simulink model "EHB_MOTOR_r2018b"  (R2018b)
settings: Solver=FixedStepDiscrete  StartTime=0.0  StopTime=0.2  FixedStep=0.0001  RelTol=1e-3  EnableMultiTasking=on
undefined symbols (not defined in the file): CAN_EHB_VCU0x125, CAN_EHB_VCU0x126, CAN_id0x120_Data, Cos_Table, Cos_Table1, EHB_DTC_status, Sin_BreakPoint, Sin_BreakPoint1, Sin_Table, Sin_Table1
libraries: simulink x30
(part 2 of 7)

== system EHB_MOTOR_r2018b/EPB_CTRL/Subsystem1 ==
  Trigger : TriggerPort  TriggerType=function-call  VariantControl=Variant  PortDimensions=1
  Bus Creator : BusCreator  Inputs=11
  Data Store Memory11 : DataStoreMemory  DataStoreName=EPB_vBAT_AD  ReadBeforeWriteMsg=warning  WriteAfterWriteMsg=warning  WriteAfterReadMsg=warning  ShowAdditionalParam=off  OutDataTypeStr=uint16
      settings: RTWStateStorageClass=ExportedGlobal
  Data Store Memory12 : DataStoreMemory  DataStoreName=EPB1_Temp_AD  ReadBeforeWriteMsg=warning  WriteAfterWriteMsg=warning  WriteAfterReadMsg=warning  ShowAdditionalParam=off  OutDataTypeStr=uint16
      settings: RTWStateStorageClass=ExportedGlobal
  Data Store Memory13 : DataStoreMemory  DataStoreName=EPB_APBSwitch2_AD  ReadBeforeWriteMsg=warning  WriteAfterWriteMsg=warning  WriteAfterReadMsg=warning  ShowAdditionalParam=off  OutDataTypeStr=uint16
      settings: RTWStateStorageClass=ExportedGlobal
  Data Store Memory14 : DataStoreMemory  DataStoreName=EPB_7181PreDriver1_AD  ReadBeforeWriteMsg=warning  WriteAfterWriteMsg=warning  WriteAfterReadMsg=warning  ShowAdditionalParam=off  OutDataTypeStr=uint16
      settings: RTWStateStorageClass=ExportedGlobal
  Data Store Memory15 : DataStoreMemory  DataStoreName=EPB2_Temp_AD  ReadBeforeWriteMsg=warning  WriteAfterWriteMsg=warning  WriteAfterReadMsg=warning  ShowAdditionalParam=off  OutDataTypeStr=uint16
      settings: RTWStateStorageClass=ExportedGlobal
  Data Store Memory17 : DataStoreMemory  DataStoreName=EPB_APBSwitch3_AD  ReadBeforeWriteMsg=warning  WriteAfterWriteMsg=warning  WriteAfterReadMsg=warning  ShowAdditionalParam=off  OutDataTypeStr=uint16
      settings: RTWStateStorageClass=ExportedGlobal
  Data Store Memory18 : DataStoreMemory  DataStoreName=EPB_APBSwitch4_AD  ReadBeforeWriteMsg=warning  WriteAfterWriteMsg=warning  WriteAfterReadMsg=warning  ShowAdditionalParam=off  OutDataTypeStr=uint16
      settings: RTWStateStorageClass=ExportedGlobal
  Data Store Memory19 : DataStoreMemory  DataStoreName=EPB2_Current_AD  ReadBeforeWriteMsg=warning  WriteAfterWriteMsg=warning  WriteAfterReadMsg=warning  ShowAdditionalParam=off  OutDataTypeStr=uint16
      settings: RTWStateStorageClass=ExportedGlobal
  Data Store Memory20 : DataStoreMemory  DataStoreName=EPB_APBSwitch1_AD  ReadBeforeWriteMsg=warning  WriteAfterWriteMsg=warning  WriteAfterReadMsg=warning  ShowAdditionalParam=off  OutDataTypeStr=uint16
      settings: RTWStateStorageClass=ExportedGlobal
  Data Store Memory21 : DataStoreMemory  DataStoreName=EPB1_Current_AD  ReadBeforeWriteMsg=warning  WriteAfterWriteMsg=warning  WriteAfterReadMsg=warning  ShowAdditionalParam=off  OutDataTypeStr=uint16
      settings: RTWStateStorageClass=ExportedGlobal
  Data Store Memory22 : DataStoreMemory  DataStoreName=EPB_7181PreDriver2_AD  ReadBeforeWriteMsg=warning  WriteAfterWriteMsg=warning  WriteAfterReadMsg=warning  ShowAdditionalParam=off  OutDataTypeStr=uint16
      settings: RTWStateStorageClass=ExportedGlobal
  Data Store Read11 : DataStoreRead  DataStoreName=EPB_vBAT_AD  DataStoreElements=EPB_vBAT_AD
  Data Store Read12 : DataStoreRead  DataStoreName=EPB1_Temp_AD  DataStoreElements=EPB1_Temp_AD
  Data Store Read13 : DataStoreRead  DataStoreName=EPB_APBSwitch2_AD  DataStoreElements=EPB_APBSwitch2_AD
  Data Store Read14 : DataStoreRead  DataStoreName=EPB_7181PreDriver1_AD  DataStoreElements=EPB_7181PreDriver1_AD
  Data Store Read15 : DataStoreRead  DataStoreName=EPB2_Temp_AD  DataStoreElements=EPB2_Temp_AD
  Data Store Read17 : DataStoreRead  DataStoreName=EPB_APBSwitch3_AD  DataStoreElements=EPB_APBSwitch3_AD
  Data Store Read18 : DataStoreRead  DataStoreName=EPB_APBSwitch4_AD  DataStoreElements=EPB_APBSwitch4_AD
  Data Store Read19 : DataStoreRead  DataStoreName=EPB2_Current_AD  DataStoreElements=EPB2_Current_AD
  Data Store Read20 : DataStoreRead  DataStoreName=EPB_APBSwitch1_AD  DataStoreElements=EPB_APBSwitch1_AD
  Data Store Read21 : DataStoreRead  DataStoreName=EPB1_Current_AD  DataStoreElements=EPB1_Current_AD
  Data Store Read22 : DataStoreRead  DataStoreName=EPB_7181PreDriver2_AD  DataStoreElements=EPB_7181PreDriver2_AD
  EPB_interface : Subsystem
  EPB_INPUTBUS : Outport
  wires:
  Data Store Read21/1 -> EPB_interface/2(EPB1_Current_AD)
  Data Store Read17/1 -> EPB_interface/6(EPB_APBSwitch3_AD)
  Data Store Read14/1 -> EPB_interface/11(EPB_7181PreDriver1_AD)
  Data Store Read13/1 -> EPB_interface/10(EPB_7181PreDriver2_AD)
  EPB_interface/9(EPB_APBSwitch2_filtered) -> Bus Creator/9  "EPB_7181PreDriver2_filtered"
  Data Store Read19/1 -> EPB_interface/3(EPB2_Current_AD)
  Data Store Read12/1 -> EPB_interface/4(EPB1_Temp_AD)
  Data Store Read22/1 -> EPB_interface/9(EPB_APBSwitch2_AD)
  Data Store Read15/1 -> EPB_interface/5(EPB2_Temp_AD)
  Data Store Read20/1 -> EPB_interface/8(EPB_APBSwitch1_AD)
  EPB_interface/7(EPB_APBSwitch4_filtered) -> Bus Creator/7  "EPB_APBSwitch4_filtered"
  EPB_interface/11(EPB_7181PreDriver1_filtered) -> Bus Creator/11  "EPB_7181PreDriver1_filtered"
  EPB_interface/4(EPB1_Temp) -> Bus Creator/4  "EPB1_Temp"
  EPB_interface/3(EPB2_Current_filtered) -> Bus Creator/3  "EPB2_Current_filtered"
  Data Store Read11/1 -> EPB_interface/1(EPB_vBAT_AD)
  EPB_interface/2(EPB1_Current_filtered) -> Bus Creator/2  "EPB1_Current_filtered"
  Data Store Read18/1 -> EPB_interface/7(EPB_APBSwitch4_AD)
  EPB_interface/6(EPB_APBSwitch3_filtered) -> Bus Creator/6  "EPB_APBSwitch3_filtered"
  EPB_interface/5(EPB2_Temp) -> Bus Creator/5  "EPB2_Temp"
  EPB_interface/1(EPB_vBAT_filtered) -> Bus Creator/1  "EPB_vBAT_filtered"
  EPB_interface/10(EPB_7181PreDriver2_filtered) -> Bus Creator/10  "EPB_APBSwitch2_filtered"
  EPB_interface/8(EPB_APBSwitch1_filtered) -> Bus Creator/8  "EPB_APBSwitch1_filtered"
  Bus Creator/1 -> EPB_INPUTBUS/1

== system EHB_MOTOR_r2018b/EHB_MOTOR_PRO/DIAG/5vDiag ==
  note: 20ms
  note: 5v输出异常
  5vVoltage : Inport
  Chart : Stateflow chart  TreatAsAtomicUnit=on
  Subsystem : Subsystem
  5vErr : Outport
  wires:
  5vVoltage/1 -> Subsystem/1(In1)
  Subsystem/1(Out1) -> 5vErr/1
  Chart/1(task_20ms()) -> Subsystem/Trigger

== system EHB_MOTOR_r2018b/EHB_MOTOR_PRO/DIAG/AngleSensorDiag ==
  note: 角度传感器缺少标定
  note: 角度传感器没有信号
  note: 200ms
  note: 角度传感器信号超限故障
  note: 200ms
  note: 200ms
  AngleSensorSignal : Inport
  AngleSensorCalFlag : Inport  Port=2
  Chart : Stateflow chart  TreatAsAtomicUnit=on
  Chart1 : Stateflow chart  TreatAsAtomicUnit=on
  Chart2 : Stateflow chart  TreatAsAtomicUnit=on
  Subsystem : Subsystem
  Subsystem1 : Subsystem
  Subsystem2 : Subsystem
  AngleSensorSignalOverride : Outport
  AngleSensorSignalLost : Outport  Port=2
  AngleSensorNoCal : Outport  Port=3
  wires:
  Subsystem/1(Out1) -> AngleSensorSignalOverride/1
  Chart/1(task_200ms()) -> Subsystem/Trigger
  Chart1/1(task_200ms()) -> Subsystem1/Trigger
  Subsystem1/1(Out1) -> AngleSensorSignalLost/1
  AngleSensorSignal/1 -> Subsystem1/1(In1), Subsystem/1(In1)
  Subsystem2/1(Out1) -> AngleSensorNoCal/1
  Chart2/1(task_200ms()) -> Subsystem2/Trigger
  AngleSensorCalFlag/1 -> Subsystem2/1(In1)

== system EHB_MOTOR_r2018b/EHB_MOTOR_PRO/DIAG/BusOffDiag ==
  note: 控制器内部故障
  In1 : Inport
  Ground : Ground
  Terminator : Terminator
  BusOffErr : Outport
  wires:
  In1/1 -> Terminator/1
  Ground/1 -> BusOffErr/1

== system EHB_MOTOR_r2018b/EHB_MOTOR_PRO/DIAG/CANCommDiag ==
  note: CAN收发模块故障
  In1 : Inport
  Ground : Ground
  Terminator : Terminator
  CANCommErr : Outport
  wires:
  In1/1 -> Terminator/1
  Ground/1 -> CANCommErr/1

== system EHB_MOTOR_r2018b/EHB_MOTOR_PRO/DIAG/CANDataLostDiag ==
  note: CAN丢失数据
  In1 : Inport
  Ground : Ground
  Terminator : Terminator
  CANDataLostErr : Outport
  wires:
  In1/1 -> Terminator/1
  Ground/1 -> CANDataLostErr/1

== system EHB_MOTOR_r2018b/EHB_MOTOR_PRO/DIAG/Chip7189Diag ==
  note: 7189芯片故障
  note: 20ms
  Chart : Stateflow chart  TreatAsAtomicUnit=on
  Data Store Memory1 : DataStoreMemory  DataStoreName=Chip7189ErrFlag  ReadBeforeWriteMsg=warning  WriteAfterWriteMsg=warning  WriteAfterReadMsg=warning  ShowAdditionalParam=off  OutDataTypeStr=uint8
      settings: RTWStateStorageClass=ExportedGlobal
  Data Store Read2 : DataStoreRead  DataStoreName=Chip7189ErrFlag  DataStoreElements=Chip7189ErrFlag
  Subsystem : Subsystem
  Chip7189_err : Outport
  wires:
  Chart/1(task_20ms()) -> Subsystem/Trigger
  Subsystem/1(Out1) -> Chip7189_err/1
  Data Store Read2/1 -> Subsystem/1(In1)

== system EHB_MOTOR_r2018b/EHB_MOTOR_PRO/DIAG/CurrentSensorDiag ==
  note: 200ms
  note: U相电流传感器故障
  note: 200ms
  note: V相电流传感器故障
  note: 200ms
  note: W相电流传感器故障
  CurrentSensorU : Inport
  CurrentSensorV : Inport  Port=2
  CurrentSensorW : Inport  Port=3
  Chart : Stateflow chart  TreatAsAtomicUnit=on
  Chart1 : Stateflow chart  TreatAsAtomicUnit=on
  Chart2 : Stateflow chart  TreatAsAtomicUnit=on
  Subsystem : Subsystem
  Subsystem1 : Subsystem
  Subsystem2 : Subsystem
  CurrentSensorUOverride : Outport
  CurrentSensorVOverride : Outport  Port=2
  CurrentSensorWOverride : Outport  Port=3
  wires:
  CurrentSensorU/1 -> Subsystem/1(In1)
  Subsystem/1(Out1) -> CurrentSensorUOverride/1
  Chart/1(task_200ms()) -> Subsystem/Trigger
  Chart1/1(task_200ms()) -> Subsystem1/Trigger
  Subsystem1/1(Out1) -> CurrentSensorVOverride/1
  CurrentSensorV/1 -> Subsystem1/1(In1)
  CurrentSensorW/1 -> Subsystem2/1(In1)
  Subsystem2/1(Out1) -> CurrentSensorWOverride/1
  Chart2/1(task_200ms()) -> Subsystem2/Trigger

== system EHB_MOTOR_r2018b/EHB_MOTOR_PRO/DIAG/EHBDiag ==
  note: EHB电源电压过高
  note: 200ms
  note: EHB电源电压过低
  EHBVoltage : Inport
  Chart : Stateflow chart  TreatAsAtomicUnit=on
  Subsystem : Subsystem
  EHBVoltageLow1 : Outport
  EHBVoltageLow2 : Outport  Port=2
  EHBVoltageHigh1 : Outport  Port=3
  EHBVoltageHigh2 : Outport  Port=4
  wires:
  EHBVoltage/1 -> Subsystem/1(In1)
  Subsystem/1(EHBVoltageLow1) -> EHBVoltageLow1/1
  Chart/1(task_200ms()) -> Subsystem/Trigger
  Subsystem/3(EHBVoltageHigh1) -> EHBVoltageHigh1/1
  Subsystem/2(EHBVoltageLow2) -> EHBVoltageLow2/1
  Subsystem/4(EHBVoltageHigh2) -> EHBVoltageHigh2/1

== system EHB_MOTOR_r2018b/EHB_MOTOR_PRO/DIAG/KL15VoltageDiag ==
  note: KL15电压过低
  note: 200ms
  note: KL15电压过高
  KL15Voltage : Inport
  Chart : Stateflow chart  TreatAsAtomicUnit=on
  Subsystem : Subsystem
  KL15VoltageLow : Outport
  KL15VoltageHigh : Outport  Port=2
  wires:
  Subsystem/2(Out2) -> KL15VoltageHigh/1
  Chart/1(task_200ms()) -> Subsystem/Trigger
  Subsystem/1(Out1) -> KL15VoltageLow/1
  KL15Voltage/1 -> Subsystem/1(In1)

== system EHB_MOTOR_r2018b/EHB_MOTOR_PRO/DIAG/LogicVoltageDiag ==
  note: 12VLogic电源电压过高
  note: 200ms
  note: 12VLogic电源电压过低
  LogicVoltage : Inport
  Chart : Stateflow chart  TreatAsAtomicUnit=on
  Subsystem : Subsystem
  LogicVoltageLow : Outport
  LogicVoltageHigh : Outport  Port=2
  wires:
  LogicVoltage/1 -> Subsystem/1(In1)
  Subsystem/1(Out1) -> LogicVoltageLow/1
  Chart/1(task_200ms()) -> Subsystem/Trigger
  Subsystem/2(Out2) -> LogicVoltageHigh/1

== system EHB_MOTOR_r2018b/EHB_MOTOR_PRO/DIAG/MotLockDiag ==
  In1 : Inport
  Abs : Abs
  Abs1 : Abs
  Abs2 : Abs
  Bus Selector : BusSelector  OutputSignals=Feedback.TEMP_DELAY.EHB_Mot_length,AI_BUS.EHB_iU_filtered,AI_BUS.EHB_iV_filtered,AI_BUS.EHB_iW_filtered
  Constant : Constant  Value=2
  Constant1 : Constant  Value=70
  Constant2 : Constant  Value=70
  Constant3 : Constant  Value=70
  Constant4 : Constant  Value=0  OutDataTypeStr=uint8
  Data Store Memory1 : DataStoreMemory  DataStoreName=tiMotLocked_C  ReadBeforeWriteMsg=warning  WriteAfterWriteMsg=warning  WriteAfterReadMsg=warning  ShowAdditionalParam=off  OutDataTypeStr=uint16
      settings: RTWStateStorageClass=ExportedGlobal
  Data Store Read : DataStoreRead  DataStoreName=tiMotLocked_C  DataStoreElements=tiMotLocked_C
  ErrorSignalCount : Stateflow chart  TreatAsAtomicUnit=on
  Logical Operator : Logic  Operator=OR  Inputs=3  AllPortsSameDT=off  OutDataTypeStr=boolean
  Logical Operator1 : Logic  AllPortsSameDT=off  OutDataTypeStr=boolean
  Relational Operator : RelationalOperator  Operator=<  OutDataTypeStr=boolean  RndMeth=Simplest
  Relational Operator1 : RelationalOperator  Operator=>  OutDataTypeStr=boolean  RndMeth=Simplest
  Relational Operator2 : RelationalOperator  Operator=>  OutDataTypeStr=boolean  RndMeth=Simplest
  Relational Operator3 : RelationalOperator  Operator=>  OutDataTypeStr=boolean  RndMeth=Simplest
  Mot_locked_err : Outport
  wires:
  In1/1 -> Bus Selector/1
  Bus Selector/1 -> Relational Operator/1  "<EHB_Mot_length>"
  Constant/1 -> Relational Operator/2
  Constant1/1 -> Relational Operator1/2
  Bus Selector/2 -> Abs/1  "<EHB_iU_filtered>"
  Constant2/1 -> Relational Operator2/2
  Constant3/1 -> Relational Operator3/2
  Bus Selector/4 -> Abs2/1  "<EHB_iW_filtered>"
  Bus Selector/3 -> Abs1/1  "<EHB_iV_filtered>"
  Relational Operator1/1 -> Logical Operator/1
  Relational Operator2/1 -> Logical Operator/2
  Relational Operator3/1 -> Logical Operator/3
  Logical Operator/1 -> Logical Operator1/2
  Relational Operator/1 -> Logical Operator1/1
  Logical Operator1/1 -> ErrorSignalCount/1(Mot_locked)
  Abs/1 -> Relational Operator1/1
  Abs1/1 -> Relational Operator2/1
  Abs2/1 -> Relational Operator3/1
  Constant4/1 -> ErrorSignalCount/3(Recover)
  ErrorSignalCount/1(Mot_locked_err) -> Mot_locked_err/1
  Data Store Read/1 -> ErrorSignalCount/2(tiMotLocked_C)

== system EHB_MOTOR_r2018b/EHB_MOTOR_PRO/DIAG/MotorDiag ==
  note: 200ms
  note: 电机回路故障
  note: 200ms
  note: 电机过温
  note: 电机过流故障
  note: 200ms
  MotorCircuitCurrent : Inport
  Motor_PWMout : Inport  Port=2
  MotorTemp : Inport  Port=3
  MotorCurrent : Inport  Port=4
  Chart : Stateflow chart  TreatAsAtomicUnit=on
  Chart1 : Stateflow chart  TreatAsAtomicUnit=on
  Chart2 : Stateflow chart  TreatAsAtomicUnit=on
  Subsystem : Subsystem
  Subsystem1 : Subsystem
  Subsystem2 : Subsystem
  MotorCircuitCurrentOverride : Outport
  MotorTempOverride : Outport  Port=2
  MotorCurrentOverride : Outport  Port=3
  wires:
  Subsystem1/1(Out1) -> MotorTempOverride/1
  Chart1/1(task_200ms()) -> Subsystem1/Trigger
  Chart/1(task_200ms()) -> Subsystem/Trigger
  Subsystem/1(Out1) -> MotorCircuitCurrentOverride/1
  MotorCircuitCurrent/1 -> Subsystem/1(In1)
  MotorTemp/1 -> Subsystem1/1(In1)
  MotorCurrent/1 -> Subsystem2/1(In1)
  Subsystem2/1(Out1) -> MotorCurrentOverride/1
  Chart2/1(task_200ms()) -> Subsystem2/Trigger
  Motor_PWMout/1 -> Subsystem/2(Motor_PWMout)

== system EHB_MOTOR_r2018b/EHB_MOTOR_PRO/DIAG/PWMCircuitDiag ==
  note: PWM波发送电路故障
  In1 : Inport
  Ground : Ground
  Terminator : Terminator
  PWMCircuitErr : Outport
  wires:
  In1/1 -> Terminator/1
  Ground/1 -> PWMCircuitErr/1

== system EHB_MOTOR_r2018b/EHB_MOTOR_PRO/DIAG/PressureSensorDiag ==
  note: 200ms
  note: 200ms
  note: 压力跟随故障
  note: 200ms
  note: 压力传感器故障
  note: 压力传感器缺少标定
  VCU_Brake_AimPressure : Inport
  EHB_actPresure_filtered : Inport  Port=2
  EHB_Presure_ADC : Inport  Port=3
  PressureSensorCalFlag : Inport  Port=4
  Chart : Stateflow chart  TreatAsAtomicUnit=on
  Chart1 : Stateflow chart  TreatAsAtomicUnit=on
  Chart2 : Stateflow chart  TreatAsAtomicUnit=on
  Subsystem : Subsystem
  Subsystem1 : Subsystem
  Subsystem2 : Subsystem
  PressureFlowERR1 : Outport
  PressureFlowERR2 : Outport  Port=2
  PressureSensorERR : Outport  Port=3
  PressureSensorNoCal : Outport  Port=4
  wires:
  Chart2/1(task_200ms()) -> Subsystem2/Trigger
  Subsystem2/1(Out1) -> PressureSensorNoCal/1
  EHB_actPresure_filtered/1 -> Subsystem/2(EHB_actPresure_filtered)
  Subsystem1/1(Out1) -> PressureSensorERR/1
  Chart1/1(task_200ms()) -> Subsystem1/Trigger
  Chart/1(task_200ms()) -> Subsystem/Trigger
  Subsystem/1(Out1) -> PressureFlowERR1/1
  PressureSensorCalFlag/1 -> Subsystem2/1(In1)
  VCU_Brake_AimPressure/1 -> Subsystem/1(VCU_Brake_AimPressure)
  Subsystem/2(Out2) -> PressureFlowERR2/1
  EHB_Presure_ADC/1 -> Subsystem1/1(EHB_Presure_ADC)

== system EHB_MOTOR_r2018b/EHB_MOTOR_PRO/DIAG/RespondOvertimeDiag ==
  note: 响应超时故障
  In1 : Inport
  Ground : Ground
  Terminator : Terminator
  Chip7189_err : Outport
  wires:
  Ground/1 -> Chip7189_err/1
  In1/1 -> Terminator/1

== system EHB_MOTOR_r2018b/EHB_MOTOR_PRO/DIAG/SpeedSensorDiag ==
  note: 200ms
  note: 轮速传感器信号电压异常
  SpeedSensor : Inport
  Chart : Stateflow chart  TreatAsAtomicUnit=on
  Subsystem : Subsystem
  SpeedSensorOverride : Outport
  wires:
  SpeedSensor/1 -> Subsystem/1(In1)
  Chart/1(task_200ms()) -> Subsystem/Trigger
  Subsystem/1(Out1) -> SpeedSensorOverride/1

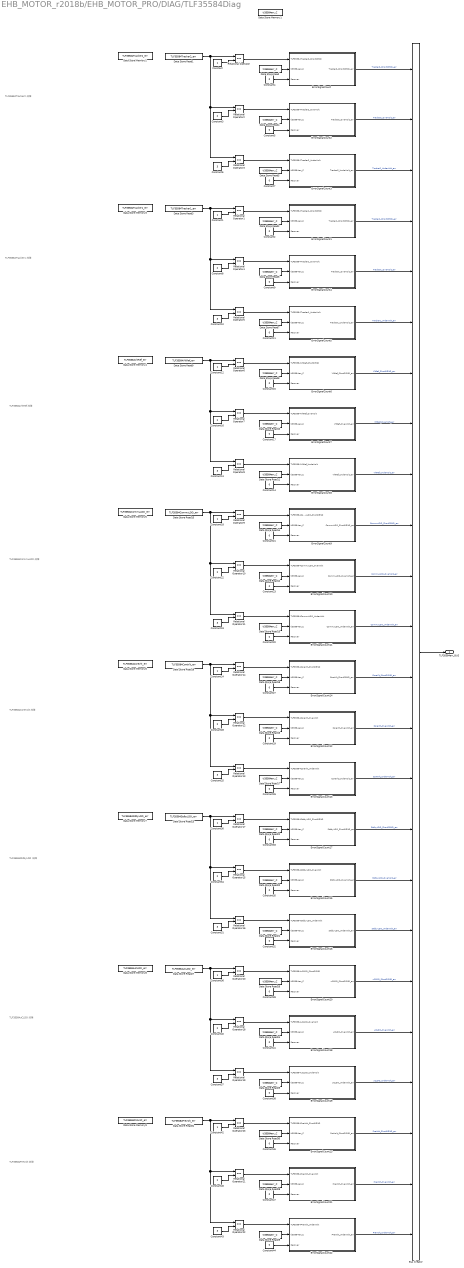
== system EHB_MOTOR_r2018b/EHB_MOTOR_PRO/DIAG/TLF35584Diag ==
  note: TLF35584Tracker2故障
  note: TLF35584Tracker1故障
  note: TLF35584VltRef故障
  note: TLF35584CommuLDO故障
  note: TLF35584CoreVolt故障
  note: TLF35584StdbyLDO故障
  note: TLF35584uCLDO故障
  note: TLF35584PreVolt故障
  Bus Creator : BusCreator  Inputs=24
  Constant{,1,12,18,24,30,36,42} (8 alike) : Constant
  Constant{6,10,13,19,25,31,37,43} (8 alike) : Constant  Value=3
  Constant{2,4..5,7,9,11,14..15,17,20..21,23,26..27,29,32..33,35,38..39,41,44..45,47} (24 alike) : Constant  Value=0  OutDataTypeStr=uint8
  Constant{3,8,16,22,28,34,40,46} (8 alike) : Constant  Value=2
  Data Store Memory1 : DataStoreMemory  DataStoreName=ti35584err_C  ReadBeforeWriteMsg=warning  WriteAfterWriteMsg=warning  WriteAfterReadMsg=warning  ShowAdditionalParam=off  OutDataTypeStr=uint16
      settings: RTWStateStorageClass=ExportedGlobal
  Data Store Memory2 : DataStoreMemory  DataStoreName=TLF35584Tracker2_err  ReadBeforeWriteMsg=warning  WriteAfterWriteMsg=warning  WriteAfterReadMsg=warning  ShowAdditionalParam=off  OutDataTypeStr=uint8
      settings: RTWStateStorageClass=ExportedGlobal
  Data Store Memory3 : DataStoreMemory  DataStoreName=TLF35584Tracker1_err  ReadBeforeWriteMsg=warning  WriteAfterWriteMsg=warning  WriteAfterReadMsg=warning  ShowAdditionalParam=off  OutDataTypeStr=uint8
      settings: RTWStateStorageClass=ExportedGlobal
  Data Store Memory4 : DataStoreMemory  DataStoreName=TLF35584VltRef_err  ReadBeforeWriteMsg=warning  WriteAfterWriteMsg=warning  WriteAfterReadMsg=warning  ShowAdditionalParam=off  OutDataTypeStr=uint8
      settings: RTWStateStorageClass=ExportedGlobal
  Data Store Memory5 : DataStoreMemory  DataStoreName=TLF35584CommuLDO_err  ReadBeforeWriteMsg=warning  WriteAfterWriteMsg=warning  WriteAfterReadMsg=warning  ShowAdditionalParam=off  OutDataTypeStr=uint8
      settings: RTWStateStorageClass=ExportedGlobal
  Data Store Memory6 : DataStoreMemory  DataStoreName=TLF35584CoreVlt_err  ReadBeforeWriteMsg=warning  WriteAfterWriteMsg=warning  WriteAfterReadMsg=warning  ShowAdditionalParam=off  OutDataTypeStr=uint8
      settings: RTWStateStorageClass=ExportedGlobal
  Data Store Memory7 : DataStoreMemory  DataStoreName=TLF35584StdbyLDO_err  ReadBeforeWriteMsg=warning  WriteAfterWriteMsg=warning  WriteAfterReadMsg=warning  ShowAdditionalParam=off  OutDataTypeStr=uint8
      settings: RTWStateStorageClass=ExportedGlobal
  Data Store Memory8 : DataStoreMemory  DataStoreName=TLF35584uCLDO_err  ReadBeforeWriteMsg=warning  WriteAfterWriteMsg=warning  WriteAfterReadMsg=warning  ShowAdditionalParam=off  OutDataTypeStr=uint8
      settings: RTWStateStorageClass=ExportedGlobal
  Data Store Memory9 : DataStoreMemory  DataStoreName=TLF35584PreVolt_err  ReadBeforeWriteMsg=warning  WriteAfterWriteMsg=warning  WriteAfterReadMsg=warning  ShowAdditionalParam=off  OutDataTypeStr=uint8
      settings: RTWStateStorageClass=ExportedGlobal
  Data Store Read{,2,4..8,10..14,16..18,20..22,24..26,28..30} (24 alike) : DataStoreRead  DataStoreName=ti35584err_C  DataStoreElements=ti35584err_C
  Data Store Read1 : DataStoreRead  DataStoreName=TLF35584Tracker2_err  DataStoreElements=TLF35584Tracker2_err
  Data Store Read15 : DataStoreRead  DataStoreName=TLF35584CommuLDO_err  DataStoreElements=TLF35584CommuLDO_err
  Data Store Read19 : DataStoreRead  DataStoreName=TLF35584CoreVlt_err  DataStoreElements=TLF35584CoreVlt_err
  Data Store Read23 : DataStoreRead  DataStoreName=TLF35584StdbyLDO_err  DataStoreElements=TLF35584StdbyLDO_err
  Data Store Read27 : DataStoreRead  DataStoreName=TLF35584uCLDO_err  DataStoreElements=TLF35584uCLDO_err
  Data Store Read3 : DataStoreRead  DataStoreName=TLF35584Tracker1_err  DataStoreElements=TLF35584Tracker1_err
  Data Store Read31 : DataStoreRead  DataStoreName=TLF35584PreVolt_err  DataStoreElements=TLF35584PreVolt_err
  Data Store Read9 : DataStoreRead  DataStoreName=TLF35584VltRef_err  DataStoreElements=TLF35584VltRef_err
  ErrorSignalCount : Stateflow chart  TreatAsAtomicUnit=on
  ErrorSignalCount1 : Stateflow chart  TreatAsAtomicUnit=on
  ErrorSignalCount10 : Stateflow chart  TreatAsAtomicUnit=on
  ErrorSignalCount11 : Stateflow chart  TreatAsAtomicUnit=on
  ErrorSignalCount12 : Stateflow chart  TreatAsAtomicUnit=on
  ErrorSignalCount13 : Stateflow chart  TreatAsAtomicUnit=on
  ErrorSignalCount14 : Stateflow chart  TreatAsAtomicUnit=on
  ErrorSignalCount15 : Stateflow chart  TreatAsAtomicUnit=on
  ErrorSignalCount16 : Stateflow chart  TreatAsAtomicUnit=on
  ErrorSignalCount17 : Stateflow chart  TreatAsAtomicUnit=on
  ErrorSignalCount18 : Stateflow chart  TreatAsAtomicUnit=on
  ErrorSignalCount19 : Stateflow chart  TreatAsAtomicUnit=on
  ErrorSignalCount2 : Stateflow chart  TreatAsAtomicUnit=on
  ErrorSignalCount20 : Stateflow chart  TreatAsAtomicUnit=on
  ErrorSignalCount21 : Stateflow chart  TreatAsAtomicUnit=on
  ErrorSignalCount22 : Stateflow chart  TreatAsAtomicUnit=on
  ErrorSignalCount23 : Stateflow chart  TreatAsAtomicUnit=on
  ErrorSignalCount3 : Stateflow chart  TreatAsAtomicUnit=on
  ErrorSignalCount4 : Stateflow chart  TreatAsAtomicUnit=on
  ErrorSignalCount5 : Stateflow chart  TreatAsAtomicUnit=on
  ErrorSignalCount6 : Stateflow chart  TreatAsAtomicUnit=on
  ErrorSignalCount7 : Stateflow chart  TreatAsAtomicUnit=on
  ErrorSignalCount8 : Stateflow chart  TreatAsAtomicUnit=on
  ErrorSignalCount9 : Stateflow chart  TreatAsAtomicUnit=on
  Relational Operator{,1..23} (24 alike) : RelationalOperator  Operator===  OutDataTypeStr=boolean  RndMeth=Simplest
  TLF35584err_BUS : Outport
  wires:
  Data Store Read/1 -> ErrorSignalCount/2(ti35584err_C)
  Constant4/1 -> ErrorSignalCount/3(Recover)
  Data Store Read1/1 -> Relational Operator/1, Relational Operator2/1, Relational Operator3/1
  Constant/1 -> Relational Operator/2
  Relational Operator/1 -> ErrorSignalCount/1(TLF35584Tracker2_Short2GND)
  Relational Operator1/1 -> ErrorSignalCount1/1(TLF35584Tracker1_Short2GND)
  Constant1/1 -> Relational Operator1/2
  Constant2/1 -> ErrorSignalCount1/3(Recover)
  Data Store Read2/1 -> ErrorSignalCount1/2(ti35584err_C)
  Constant3/1 -> Relational Operator2/2
  Constant5/1 -> ErrorSignalCount2/3(Recover)
  Data Store Read4/1 -> ErrorSignalCount2/2(ti35584err_C)
  Relational Operator2/1 -> ErrorSignalCount2/1(TLF35584Tracker2_OverVolt)
  Constant6/1 -> Relational Operator3/2
  Relational Operator3/1 -> ErrorSignalCount3/1(TLF35584Tracker2_UnderVolt)
  Data Store Read5/1 -> ErrorSignalCount3/2(ti35584err_C)
  Constant7/1 -> ErrorSignalCount3/3(Recover)
  Constant11/1 -> ErrorSignalCount5/3(Recover)
  Data Store Read7/1 -> ErrorSignalCount5/2(ti35584err_C)
  Relational Operator5/1 -> ErrorSignalCount5/1(TLF35584Tracker1_UnderVolt)
  Constant10/1 -> Relational Operator5/2
  Relational Operator4/1 -> ErrorSignalCount4/1(TLF35584Tracker1_OverVolt)
  Data Store Read6/1 -> ErrorSignalCount4/2(ti35584err_C)
  Constant9/1 -> ErrorSignalCount4/3(Recover)
  Constant8/1 -> Relational Operator4/2
  Data Store Read3/1 -> Relational Operator5/1, Relational Operator4/1, Relational Operator1/1
  Data Store Read9/1 -> Relational Operator6/1, Relational Operator7/1, Relational Operator8/1
  Constant16/1 -> Relational Operator7/2
  Constant17/1 -> ErrorSignalCount7/3(Recover)
  Data Store Read10/1 -> ErrorSignalCount7/2(ti35584err_C)
  Relational Operator7/1 -> ErrorSignalCount7/1(TLF35584VltRef_OverVolt)
  Constant13/1 -> Relational Operator8/2
  Relational Operator8/1 -> ErrorSignalCount8/1(TLF35584VltRef_UnderVolt)
  Data Store Read11/1 -> ErrorSignalCount8/2(ti35584err_C)
  Constant14/1 -> ErrorSignalCount8/3(Recover)
  Data Store Read8/1 -> ErrorSignalCount6/2(ti35584err_C)
  Constant15/1 -> ErrorSignalCount6/3(Recover)
  Constant12/1 -> Relational Operator6/2
  Relational Operator6/1 -> ErrorSignalCount6/1(TLF35584VltRef_Short2GND)
  Relational Operator9/1 -> ErrorSignalCount9/1(TLF35584CommuLDO_Short2GND)
  Constant18/1 -> Relational Operator9/2
  Constant21/1 -> ErrorSignalCount9/3(Recover)
  Data Store Read14/1 -> ErrorSignalCount9/2(ti35584err_C)
  Constant20/1 -> ErrorSignalCount11/3(Recover)
  Data Store Read13/1 -> ErrorSignalCount11/2(ti35584err_C)
  Relational Operator11/1 -> ErrorSignalCount11/1(TLF35584CommuLDO_UnderVolt)
  Constant19/1 -> Relational Operator11/2
  Relational Operator10/1 -> ErrorSignalCount10/1(TLF35584CommuLDO_OverVolt)
  Data Store Read12/1 -> ErrorSignalCount10/2(ti35584err_C)
  Constant23/1 -> ErrorSignalCount10/3(Recover)
  Constant22/1 -> Relational Operator10/2
  Data Store Read15/1 -> Relational Operator11/1, Relational Operator10/1, Relational Operator9/1
  Data Store Read19/1 -> Relational Operator14/1, Relational Operator13/1, Relational Operator12/1
  Constant28/1 -> Relational Operator12/2
  Constant29/1 -> ErrorSignalCount12/3(Recover)
  Data Store Read16/1 -> ErrorSignalCount12/2(ti35584err_C)
  Relational Operator12/1 -> ErrorSignalCount12/1(TLF35584CoreVlt_OverVolt)
  Constant25/1 -> Relational Operator13/2
  Relational Operator13/1 -> ErrorSignalCount13/1(TLF35584CoreVlt_UnderVolt)
  Data Store Read17/1 -> ErrorSignalCount13/2(ti35584err_C)
  Constant26/1 -> ErrorSignalCount13/3(Recover)
  Data Store Read18/1 -> ErrorSignalCount14/2(ti35584err_C)
  Constant27/1 -> ErrorSignalCount14/3(Recover)
  Constant24/1 -> Relational Operator14/2
  Relational Operator14/1 -> ErrorSignalCount14/1(TLF35584CoreVlt_Short2GND)
  Relational Operator17/1 -> ErrorSignalCount17/1(TLF35584StdbyLDO_Short2GND)
  Constant30/1 -> Relational Operator17/2
  Constant33/1 -> ErrorSignalCount17/3(Recover)
  Data Store Read22/1 -> ErrorSignalCount17/2(ti35584err_C)
  Constant32/1 -> ErrorSignalCount16/3(Recover)
  Data Store Read21/1 -> ErrorSignalCount16/2(ti35584err_C)
  Relational Operator16/1 -> ErrorSignalCount16/1(TLF35584StdbyLDO_UnderVolt)
  Constant31/1 -> Relational Operator16/2
  Relational Operator15/1 -> ErrorSignalCount15/1(TLF35584StdbyLDO_OverVolt)
  Data Store Read20/1 -> ErrorSignalCount15/2(ti35584err_C)
  Constant35/1 -> ErrorSignalCount15/3(Recover)
  Constant34/1 -> Relational Operator15/2
  Data Store Read23/1 -> Relational Operator16/1, Relational Operator15/1, Relational Operator17/1
  Data Store Read27/1 -> Relational Operator20/1, Relational Operator19/1, Relational Operator18/1
  Constant40/1 -> Relational Operator18/2
  Constant41/1 -> ErrorSignalCount18/3(Recover)
  Data Store Read24/1 -> ErrorSignalCount18/2(ti35584err_C)
  Relational Operator18/1 -> ErrorSignalCount18/1(TLF35584uCLDO_OverVolt)
  Constant37/1 -> Relational Operator19/2
  Relational Operator19/1 -> ErrorSignalCount19/1(TLF35584uCLDO_UnderVolt)
  Data Store Read25/1 -> ErrorSignalCount19/2(ti35584err_C)
  Constant38/1 -> ErrorSignalCount19/3(Recover)
  Data Store Read26/1 -> ErrorSignalCount20/2(ti35584err_C)
  Constant39/1 -> ErrorSignalCount20/3(Recover)
  Constant36/1 -> Relational Operator20/2
  Relational Operator20/1 -> ErrorSignalCount20/1(TLF35584uCLDO_Short2GND)
  Relational Operator23/1 -> ErrorSignalCount23/1(TLF35584PreVolt_Short2GND)
  Constant42/1 -> Relational Operator23/2
  Constant45/1 -> ErrorSignalCount23/3(Recover)
  Data Store Read30/1 -> ErrorSignalCount23/2(ti35584err_C)
  Constant44/1 -> ErrorSignalCount22/3(Recover)
  Data Store Read29/1 -> ErrorSignalCount22/2(ti35584err_C)
  Relational Operator22/1 -> ErrorSignalCount22/1(TLF35584PreVolt_UnderVolt)
  Constant43/1 -> Relational Operator22/2
  Relational Operator21/1 -> ErrorSignalCount21/1(TLF35584PreVolt_OverVolt)
  Data Store Read28/1 -> ErrorSignalCount21/2(ti35584err_C)
  Constant47/1 -> ErrorSignalCount21/3(Recover)
  Constant46/1 -> Relational Operator21/2
  Data Store Read31/1 -> Relational Operator22/1, Relational Operator21/1, Relational Operator23/1
  ErrorSignalCount/1(Tracker2_Short2GND_err) -> Bus Creator/1  "Tracker2_Short2GND_err"
  ErrorSignalCount2/1(Tracker2_OverVolt_err) -> Bus Creator/2  "Tracker2_OverVolt_err"
  ErrorSignalCount3/1(Tracker2_UnderVolt_err) -> Bus Creator/3  "Tracker2_UnderVolt_err"
  ErrorSignalCount1/1(Tracker1_Short2GND_err) -> Bus Creator/4  "Tracker1_Short2GND_err"
  ErrorSignalCount4/1(Tracker1_OverVolt_err) -> Bus Creator/5  "Tracker1_OverVolt_err"
  ErrorSignalCount5/1(Tracker1_UnderVolt_err) -> Bus Creator/6  "Tracker1_UnderVolt_err"
  ErrorSignalCount6/1(VltRef_Short2GND_err) -> Bus Creator/7  "VltRef_Short2GND_err"
  ErrorSignalCount7/1(VltRef_OverVolt_err) -> Bus Creator/8  "VltRef_OverVolt_err"
  ErrorSignalCount8/1(VltRef_UnderVolt_err) -> Bus Creator/9  "VltRef_UnderVolt_err"
  ErrorSignalCount9/1(CommuLDO_Short2GND_err) -> Bus Creator/10  "CommuLDO_Short2GND_err"
  ErrorSignalCount10/1(CommuLDO_OverVolt_err) -> Bus Creator/11  "CommuLDO_OverVolt_err"
  ErrorSignalCount11/1(CommuLDO_UnderVolt_err) -> Bus Creator/12  "CommuLDO_UnderVolt_err"
  ErrorSignalCount14/1(CoreVlt_Short2GND_err) -> Bus Creator/13  "CoreVlt_Short2GND_err"
  ErrorSignalCount12/1(CoreVlt_OverVolt_err) -> Bus Creator/14  "CoreVlt_OverVolt_err"
  ErrorSignalCount13/1(CoreVlt_UnderVolt_err) -> Bus Creator/15  "CoreVlt_UnderVolt_err"
  ErrorSignalCount17/1(StdbyLDO_Short2GND_err) -> Bus Creator/16  "StdbyLDO_Short2GND_err"
  ErrorSignalCount15/1(StdbyLDO_OverVolt_err) -> Bus Creator/17  "StdbyLDO_OverVolt_err"
  ErrorSignalCount16/1(StdbyLDO_UnderVolt_err) -> Bus Creator/18  "StdbyLDO_UnderVolt_err"
  ErrorSignalCount20/1(uCLDO_Short2GND_err) -> Bus Creator/19  "uCLDO_Short2GND_err"
  ErrorSignalCount18/1(uCLDO_OverVolt_err) -> Bus Creator/20  "uCLDO_OverVolt_err"
  ErrorSignalCount19/1(uCLDO_UnderVolt_err) -> Bus Creator/21  "uCLDO_UnderVolt_err"
  ErrorSignalCount23/1(PreVolt_Short2GND_err) -> Bus Creator/22  "PreVolt_Short2GND_err"
  ErrorSignalCount21/1(PreVolt_OverVolt_err) -> Bus Creator/23  "PreVolt_OverVolt_err"
  ErrorSignalCount22/1(PreVolt_UnderVolt_err) -> Bus Creator/24  "PreVolt_UnderVolt_err"
  Bus Creator/1 -> TLF35584err_BUS/1

== system EHB_MOTOR_r2018b/EHB_MOTOR_PRO/DIAG/TempDiag ==
  note: 200ms
  note: 温度传感器故障
  TempSensor : Inport
  Chart : Stateflow chart  TreatAsAtomicUnit=on
  Subsystem1 : Subsystem
  TempSensorOverride : Outport
  wires:
  Subsystem1/1(Out1) -> TempSensorOverride/1
  TempSensor/1 -> Subsystem1/1(In1)
  Chart/1(task_200ms()) -> Subsystem1/Trigger

== system EHB_MOTOR_r2018b/EHB_MOTOR_PRO/DIAG/UDS_interface ==
  DiagBUS : Inport
  Bus Selector : BusSelector  OutputSignals=EHBVoltageLow2
  Bus Selector1 : BusSelector  OutputSignals=EHBVoltageHigh2
  Bus Selector10 : BusSelector  OutputSignals=5vErr
  Bus Selector12 : BusSelector  OutputSignals=Chip7189_err
  Bus Selector14 : BusSelector  OutputSignals=PressureFlowERR2
  Bus Selector2 : BusSelector  OutputSignals=TempSensorOverride
  Bus Selector3 : BusSelector  OutputSignals=PressureSensorERR
  Bus Selector4 : BusSelector  OutputSignals=CurrentSensorUOverride,CurrentSensorVOverride,CurrentSensorWOverride
  Bus Selector5 : BusSelector  OutputSignals=TLF35584err_BUS.Tracker2_Short2GND_err,TLF35584err_BUS.Tracker2_OverVolt_err,TLF35584err_BUS.Tracker2_UnderVolt_err,TLF35584err_BUS.Tracker1_Short2GND_err,TLF35584err_BUS.Tracker1_OverVolt_err,TLF35584err_BUS.Tracker1_UnderVolt_err,TLF35584err_BUS.VltRef_Short2GND_err,TLF35584err_BUS.VltRef_OverVolt_err,TLF35584err_BUS.VltRef_UnderVolt_err,TLF35584err_BUS.CommuLDO_Short2GND_err,TLF35584err_BUS.CommuLDO_OverVolt_err,TLF35584err_BUS.CommuLDO_UnderVolt_err,TLF35584err_BUS.CoreVlt_Short2GND_err,TLF35584err_BUS.CoreVlt_OverVolt_err,TLF35584err_BUS.CoreVlt_UnderVolt_err,TLF35584err_BUS.StdbyLDO_Short2GND_err,TLF35584err_BUS.StdbyLDO_OverVolt_err,TLF35584err_BUS.StdbyLDO_UnderVolt_err,TLF35584err_BUS.uCLDO_Short2GND_err,TLF35584err_BUS.uCLDO_OverVolt_err,TLF35584err_BUS.uCLDO_UnderVolt_err,TLF35584err_BUS.PreVolt_Short2GND_err,TLF35584err_BUS.PreVolt_OverVolt_err,TLF35584err_BUS.PreVolt_UnderVolt_err
  Bus Selector6 : BusSelector  OutputSignals=AngleSensorSignalOverride
  Bus Selector7 : BusSelector  OutputSignals=AngleSensorSignalLost
  Bus Selector8 : BusSelector  OutputSignals=Mot_locked_err
  Constant{,1..10,12..15} (15 alike) : Constant  Value=0
  DTC_pack : Stateflow chart  TreatAsAtomicUnit=on
  Data Store Memory2 : DataStoreMemory  DataStoreName=Clear_DTC  ReadBeforeWriteMsg=warning  WriteAfterWriteMsg=warning  WriteAfterReadMsg=warning  ShowAdditionalParam=off  OutDataTypeStr=uint8
      settings: RTWStateStorageClass=ExportedGlobal
  Data Store Read2 : DataStoreRead  DataStoreName=Clear_DTC  DataStoreElements=Clear_DTC
  Logical Operator : Logic  Operator=OR  Inputs=3  AllPortsSameDT=off  OutDataTypeStr=boolean
  EHB_DTC : Outport
  wires:
  DiagBUS/1 -> Bus Selector/1, Bus Selector1/1, Bus Selector2/1, Bus Selector3/1, Bus Selector6/1, Bus Selector7/1, Bus Selector8/1, Bus Selector10/1, Bus Selector12/1, Bus Selector14/1, Bus Selector5/1, Bus Selector4/1
  DTC_pack/1(EHB_DTC) -> EHB_DTC/1
  Bus Selector/1 -> DTC_pack/1(minBAT)  "<EHBVoltageLow2>"
  Bus Selector1/1 -> DTC_pack/2(maxBAT)  "<EHBVoltageHigh2>"
  Bus Selector2/1 -> DTC_pack/3(overTemp)  "<TempSensorOverride>"
  Bus Selector6/1 -> DTC_pack/7(errAngleSensor)  "<AngleSensorSignalOverride>"
  Bus Selector7/1 -> DTC_pack/8(noAngleSensor)  "<AngleSensorSignalLost>"
  Constant/1 -> DTC_pack/9(unCalAngleSensor)
  Constant2/1 -> DTC_pack/11(noPreSensor)
  Constant1/1 -> DTC_pack/10(errPreSensor)
  Constant3/1 -> DTC_pack/12(unCalPreSensor)
  Constant4/1 -> DTC_pack/13(errTqSensor)
  Constant5/1 -> DTC_pack/14(noTqSensor)
  Constant6/1 -> DTC_pack/15(unCalTqSensor)
  Bus Selector8/1 -> DTC_pack/16(errMotorloop)  "<Mot_locked_err>"
  Bus Selector10/1 -> DTC_pack/18(err5vOUT)  "<5vErr>"
  Bus Selector12/1 -> DTC_pack/21(errA3941)  "<Chip7189_err>"
  Bus Selector14/1 -> DTC_pack/23(errResponce)  "<PressureFlowERR2>"
  Constant7/1 -> DTC_pack/24(errCANHW)
  Constant8/1 -> DTC_pack/25(CANDataLoss)
  Constant9/1 -> DTC_pack/26(BUSOFF)
  Data Store Read2/1 -> DTC_pack/27(Clear_minBAT_req)
  Constant10/1 -> DTC_pack/4(errTempSensor)
  Logical Operator/1 -> DTC_pack/5(overCurrent)
  Bus Selector4/1 -> Logical Operator/1  "<CurrentSensorUOverride>"
  Bus Selector4/2 -> Logical Operator/2  "<CurrentSensorVOverride>"
  Bus Selector4/3 -> Logical Operator/3  "<CurrentSensorWOverride>"
  Constant12/1 -> DTC_pack/17(errPreCtl)
  Constant13/1 -> DTC_pack/19(errHSO1)
  Constant14/1 -> DTC_pack/20(errHSO2)
  Constant15/1 -> DTC_pack/22(errPWM)
  Bus Selector3/1 -> DTC_pack/6(errCurSensor)  "<PressureSensorERR>"
  Bus Selector5/1 -> DTC_pack/28(Tracker2_Short2GND_err)  "<Tracker2_Short2GND_err>"
  Bus Selector5/2 -> DTC_pack/29(Tracker2_OverVolt_err)  "<Tracker2_OverVolt_err>"
  Bus Selector5/3 -> DTC_pack/30(Tracker2_UnderVolt_err)  "<Tracker2_UnderVolt_err>"
  Bus Selector5/4 -> DTC_pack/31(Tracker1_Short2GND_err)  "<Tracker1_Short2GND_err>"
  Bus Selector5/5 -> DTC_pack/32(Tracker1_OverVolt_err)  "<Tracker1_OverVolt_err>"
  Bus Selector5/6 -> DTC_pack/33(Tracker1_UnderVolt_err)  "<Tracker1_UnderVolt_err>"
  Bus Selector5/7 -> DTC_pack/34(VltRef_Short2GND_err)  "<VltRef_Short2GND_err>"
  Bus Selector5/8 -> DTC_pack/35(VltRef_OverVolt_err)  "<VltRef_OverVolt_err>"
  Bus Selector5/9 -> DTC_pack/36(VltRef_UnderVolt_err)  "<VltRef_UnderVolt_err>"
  Bus Selector5/10 -> DTC_pack/37(CommuLDO_Short2GND_err)  "<CommuLDO_Short2GND_err>"
  Bus Selector5/11 -> DTC_pack/38(CommuLDO_OverVolt_err)  "<CommuLDO_OverVolt_err>"
  Bus Selector5/12 -> DTC_pack/39(CommuLDO_UnderVolt_err)  "<CommuLDO_UnderVolt_err>"
  Bus Selector5/13 -> DTC_pack/40(CoreVlt_Short2GND_err)  "<CoreVlt_Short2GND_err>"
  Bus Selector5/14 -> DTC_pack/41(CoreVlt_OverVolt_err)  "<CoreVlt_OverVolt_err>"
  Bus Selector5/15 -> DTC_pack/42(CoreVlt_UnderVolt_err)  "<CoreVlt_UnderVolt_err>"
  Bus Selector5/16 -> DTC_pack/43(StdbyLDO_Short2GND_err)  "<StdbyLDO_Short2GND_err>"
  Bus Selector5/17 -> DTC_pack/44(StdbyLDO_OverVolt_err)  "<StdbyLDO_OverVolt_err>"
  Bus Selector5/18 -> DTC_pack/45(StdbyLDO_UnderVolt_err)  "<StdbyLDO_UnderVolt_err>"
  Bus Selector5/19 -> DTC_pack/46(uCLDO_Short2GND_err)  "<uCLDO_Short2GND_err>"
  Bus Selector5/20 -> DTC_pack/47(uCLDO_OverVolt_err)  "<uCLDO_OverVolt_err>"
  Bus Selector5/21 -> DTC_pack/48(uCLDO_UnderVolt_err)  "<uCLDO_UnderVolt_err>"
  Bus Selector5/22 -> DTC_pack/49(PreVolt_Short2GND_err)  "<PreVolt_Short2GND_err>"
  Bus Selector5/23 -> DTC_pack/50(PreVolt_OverVolt_err)  "<PreVolt_OverVolt_err>"
  Bus Selector5/24 -> DTC_pack/51(PreVolt_UnderVolt_err)  "<PreVolt_UnderVolt_err>"

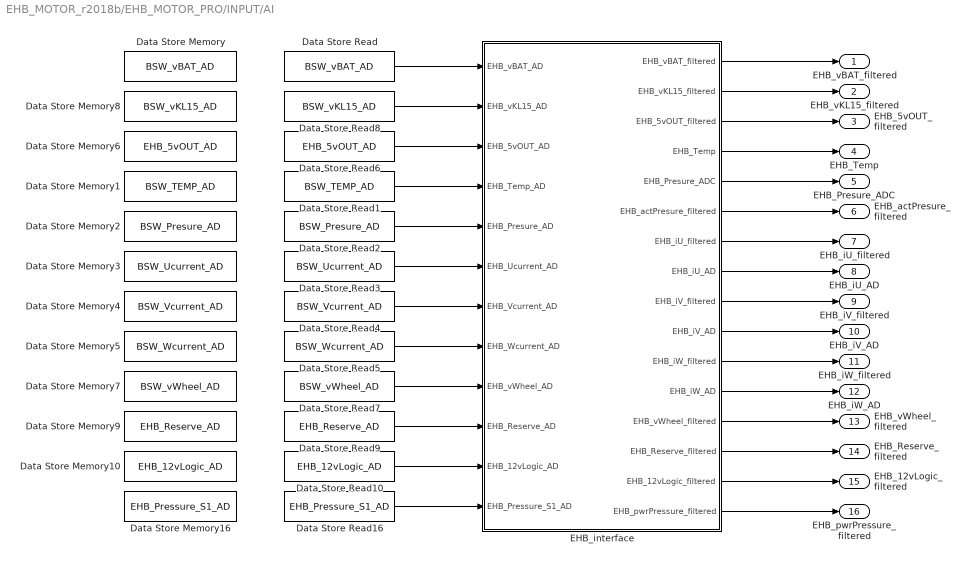
== system EHB_MOTOR_r2018b/EHB_MOTOR_PRO/INPUT/AI ==
  Data Store Memory : DataStoreMemory  DataStoreName=BSW_vBAT_AD  ReadBeforeWriteMsg=warning  WriteAfterWriteMsg=warning  WriteAfterReadMsg=warning  ShowAdditionalParam=off  OutDataTypeStr=uint16
      settings: RTWStateStorageClass=ExportedGlobal
  Data Store Memory1 : DataStoreMemory  DataStoreName=BSW_TEMP_AD  ReadBeforeWriteMsg=warning  WriteAfterWriteMsg=warning  WriteAfterReadMsg=warning  ShowAdditionalParam=off  OutDataTypeStr=uint16
      settings: RTWStateStorageClass=ExportedGlobal
  Data Store Memory10 : DataStoreMemory  DataStoreName=EHB_12vLogic_AD  ReadBeforeWriteMsg=warning  WriteAfterWriteMsg=warning  WriteAfterReadMsg=warning  ShowAdditionalParam=off  OutDataTypeStr=uint16
      settings: RTWStateStorageClass=ExportedGlobal
  Data Store Memory16 : DataStoreMemory  DataStoreName=EHB_Pressure_S1_AD  ReadBeforeWriteMsg=warning  WriteAfterWriteMsg=warning  WriteAfterReadMsg=warning  ShowAdditionalParam=off  OutDataTypeStr=uint16
      settings: RTWStateStorageClass=ExportedGlobal
  Data Store Memory2 : DataStoreMemory  DataStoreName=BSW_Presure_AD  ReadBeforeWriteMsg=warning  WriteAfterWriteMsg=warning  WriteAfterReadMsg=warning  ShowAdditionalParam=off  OutDataTypeStr=uint16
      settings: RTWStateStorageClass=ExportedGlobal
  Data Store Memory3 : DataStoreMemory  DataStoreName=BSW_Ucurrent_AD  ReadBeforeWriteMsg=warning  WriteAfterWriteMsg=warning  WriteAfterReadMsg=warning  ShowAdditionalParam=off  OutDataTypeStr=uint16
      settings: RTWStateStorageClass=ExportedGlobal
  Data Store Memory4 : DataStoreMemory  DataStoreName=BSW_Vcurrent_AD  ReadBeforeWriteMsg=warning  WriteAfterWriteMsg=warning  WriteAfterReadMsg=warning  ShowAdditionalParam=off  OutDataTypeStr=uint16
      settings: RTWStateStorageClass=ExportedGlobal
  Data Store Memory5 : DataStoreMemory  DataStoreName=BSW_Wcurrent_AD  ReadBeforeWriteMsg=warning  WriteAfterWriteMsg=warning  WriteAfterReadMsg=warning  ShowAdditionalParam=off  OutDataTypeStr=uint16
      settings: RTWStateStorageClass=ExportedGlobal
  Data Store Memory6 : DataStoreMemory  DataStoreName=EHB_5vOUT_AD  ReadBeforeWriteMsg=warning  WriteAfterWriteMsg=warning  WriteAfterReadMsg=warning  ShowAdditionalParam=off  OutDataTypeStr=uint16
      settings: RTWStateStorageClass=ExportedGlobal
  Data Store Memory7 : DataStoreMemory  DataStoreName=BSW_vWheel_AD  ReadBeforeWriteMsg=warning  WriteAfterWriteMsg=warning  WriteAfterReadMsg=warning  ShowAdditionalParam=off  OutDataTypeStr=uint16
      settings: RTWStateStorageClass=ExportedGlobal
  Data Store Memory8 : DataStoreMemory  DataStoreName=BSW_vKL15_AD  ReadBeforeWriteMsg=warning  WriteAfterWriteMsg=warning  WriteAfterReadMsg=warning  ShowAdditionalParam=off  OutDataTypeStr=uint16
      settings: RTWStateStorageClass=ExportedGlobal
  Data Store Memory9 : DataStoreMemory  DataStoreName=EHB_Reserve_AD  ReadBeforeWriteMsg=warning  WriteAfterWriteMsg=warning  WriteAfterReadMsg=warning  ShowAdditionalParam=off  OutDataTypeStr=uint16
      settings: RTWStateStorageClass=ExportedGlobal
  Data Store Read : DataStoreRead  DataStoreName=BSW_vBAT_AD  DataStoreElements=BSW_vBAT_AD
  Data Store Read1 : DataStoreRead  DataStoreName=BSW_TEMP_AD  DataStoreElements=BSW_TEMP_AD
  Data Store Read10 : DataStoreRead  DataStoreName=EHB_12vLogic_AD  DataStoreElements=EHB_12vLogic_AD
  Data Store Read16 : DataStoreRead  DataStoreName=EHB_Pressure_S1_AD  DataStoreElements=EHB_Pressure_S1_AD
  Data Store Read2 : DataStoreRead  DataStoreName=BSW_Presure_AD  DataStoreElements=BSW_Presure_AD
  Data Store Read3 : DataStoreRead  DataStoreName=BSW_Ucurrent_AD  DataStoreElements=BSW_Ucurrent_AD
  Data Store Read4 : DataStoreRead  DataStoreName=BSW_Vcurrent_AD  DataStoreElements=BSW_Vcurrent_AD
  Data Store Read5 : DataStoreRead  DataStoreName=BSW_Wcurrent_AD  DataStoreElements=BSW_Wcurrent_AD
  Data Store Read6 : DataStoreRead  DataStoreName=EHB_5vOUT_AD  DataStoreElements=EHB_5vOUT_AD
  Data Store Read7 : DataStoreRead  DataStoreName=BSW_vWheel_AD  DataStoreElements=BSW_vWheel_AD
  Data Store Read8 : DataStoreRead  DataStoreName=BSW_vKL15_AD  DataStoreElements=BSW_vKL15_AD
  Data Store Read9 : DataStoreRead  DataStoreName=EHB_Reserve_AD  DataStoreElements=EHB_Reserve_AD
  EHB_interface : Subsystem
  EHB_vBAT_filtered : Outport
  EHB_vKL15_filtered : Outport  Port=2
  EHB_5vOUT_filtered : Outport  Port=3
  EHB_Temp : Outport  Port=4
  EHB_Presure_ADC : Outport  Port=5
  EHB_actPresure_filtered : Outport  Port=6
  EHB_iU_filtered : Outport  Port=7
  EHB_iU_AD : Outport  Port=8
  EHB_iV_filtered : Outport  Port=9
  EHB_iV_AD : Outport  Port=10
  EHB_iW_filtered : Outport  Port=11
  EHB_iW_AD : Outport  Port=12
  EHB_vWheel_filtered : Outport  Port=13
  EHB_Reserve_filtered : Outport  Port=14
  EHB_12vLogic_filtered : Outport  Port=15
  EHB_pwrPressure_filtered : Outport  Port=16
  wires:
  Data Store Read8/1 -> EHB_interface/2(EHB_vKL15_AD)
  Data Store Read1/1 -> EHB_interface/4(EHB_Temp_AD)
  Data Store Read/1 -> EHB_interface/1(EHB_vBAT_AD)
  Data Store Read6/1 -> EHB_interface/3(EHB_5vOUT_AD)
  Data Store Read2/1 -> EHB_interface/5(EHB_Presure_AD)
  Data Store Read3/1 -> EHB_interface/6(EHB_Ucurrent_AD)
  Data Store Read4/1 -> EHB_interface/7(EHB_Vcurrent_AD)
  Data Store Read5/1 -> EHB_interface/8(EHB_Wcurrent_AD)
  Data Store Read7/1 -> EHB_interface/9(EHB_vWheel_AD)
  Data Store Read9/1 -> EHB_interface/10(EHB_Reserve_AD)
  Data Store Read10/1 -> EHB_interface/11(EHB_12vLogic_AD)
  Data Store Read16/1 -> EHB_interface/12(EHB_Pressure_S1_AD)
  EHB_interface/5(EHB_Presure_ADC) -> EHB_Presure_ADC/1
  EHB_interface/8(EHB_iU_AD) -> EHB_iU_AD/1
  EHB_interface/10(EHB_iV_AD) -> EHB_iV_AD/1
  EHB_interface/12(EHB_iW_AD) -> EHB_iW_AD/1
  EHB_interface/4(EHB_Temp) -> EHB_Temp/1
  EHB_interface/3(EHB_5vOUT_filtered) -> EHB_5vOUT_filtered/1
  EHB_interface/2(EHB_vKL15_filtered) -> EHB_vKL15_filtered/1
  EHB_interface/1(EHB_vBAT_filtered) -> EHB_vBAT_filtered/1
  EHB_interface/6(EHB_actPresure_filtered) -> EHB_actPresure_filtered/1
  EHB_interface/7(EHB_iU_filtered) -> EHB_iU_filtered/1
  EHB_interface/9(EHB_iV_filtered) -> EHB_iV_filtered/1
  EHB_interface/11(EHB_iW_filtered) -> EHB_iW_filtered/1
  EHB_interface/13(EHB_vWheel_filtered) -> EHB_vWheel_filtered/1
  EHB_interface/14(EHB_Reserve_filtered) -> EHB_Reserve_filtered/1
  EHB_interface/15(EHB_12vLogic_filtered) -> EHB_12vLogic_filtered/1
  EHB_interface/16(EHB_pwrPressure_filtered) -> EHB_pwrPressure_filtered/1

== system EHB_MOTOR_r2018b/EHB_MOTOR_PRO/INPUT/CAN ==
  0x120 : Stateflow chart  TreatAsAtomicUnit=on
  Data Store Memory : DataStoreMemory  DataStoreName=EHB_reqPresure  ReadBeforeWriteMsg=warning  WriteAfterWriteMsg=warning  WriteAfterReadMsg=warning  ShowAdditionalParam=off  OutDataTypeStr=single
      settings: RTWStateStorageClass=ExportedGlobal
  Data Store Memory5 : DataStoreMemory  DataStoreName=CAN_id0x120_Data  ReadBeforeWriteMsg=warning  WriteAfterWriteMsg=warning  WriteAfterReadMsg=warning  ShowAdditionalParam=off  OutDataTypeStr=uint8  Dimensions=8
      settings: RTWStateStorageClass=ExportedGlobal
  Data Store Read5 : DataStoreRead  DataStoreName=CAN_id0x120_Data  DataStoreElements=CAN_id0x120_Data(:)
  Data Store Write : DataStoreWrite  DataStoreName=EHB_reqPresure  DataStoreElements=EHB_reqPresure
  VCU_BrakingEnable : Outport
  VCU_ParkingBrakeActive : Outport  Port=2
  VCU_Brake_AimPressure : Outport  Port=3
  VCU_RollingCounter : Outport  Port=4
  VCU_Checksum : Outport  Port=5
  wires:
  0x120/1(BrakingEnable) -> VCU_BrakingEnable/1
  0x120/2(ParkingBrakeActive) -> VCU_ParkingBrakeActive/1
  0x120/3(Brake_AimPressure) -> VCU_Brake_AimPressure/1, Data Store Write/1
  0x120/4(RollingCounter) -> VCU_RollingCounter/1
  0x120/5(Checksum) -> VCU_Checksum/1
  Data Store Read5/1 -> 0x120/1(CAN_id0x120_Data)

== system EHB_MOTOR_r2018b/EHB_MOTOR_PRO/INPUT/DI ==
  Data Store Memory1 : DataStoreMemory  DataStoreName=BSW_EHB_35584err1  ReadBeforeWriteMsg=warning  WriteAfterWriteMsg=warning  WriteAfterReadMsg=warning  ShowAdditionalParam=off  OutDataTypeStr=boolean
      settings: RTWStateStorageClass=ExportedGlobal
  Data Store Memory10 : DataStoreMemory  DataStoreName=BSW_EHB_7189err1  ReadBeforeWriteMsg=warning  WriteAfterWriteMsg=warning  WriteAfterReadMsg=warning  ShowAdditionalParam=off  OutDataTypeStr=boolean
      settings: RTWStateStorageClass=ExportedGlobal
  Data Store Memory11 : DataStoreMemory  DataStoreName=BSW_EHB_7189err2  ReadBeforeWriteMsg=warning  WriteAfterWriteMsg=warning  WriteAfterReadMsg=warning  ShowAdditionalParam=off  OutDataTypeStr=boolean
      settings: RTWStateStorageClass=ExportedGlobal
  Data Store Memory12 : DataStoreMemory  DataStoreName=BSW_EHB_HID  ReadBeforeWriteMsg=warning  WriteAfterWriteMsg=warning  WriteAfterReadMsg=warning  ShowAdditionalParam=off  OutDataTypeStr=boolean
      settings: RTWStateStorageClass=ExportedGlobal
  Data Store Memory13 : DataStoreMemory  DataStoreName=BSW_EHB_AVH  ReadBeforeWriteMsg=warning  WriteAfterWriteMsg=warning  WriteAfterReadMsg=warning  ShowAdditionalParam=off  OutDataTypeStr=boolean
      settings: RTWStateStorageClass=ExportedGlobal
  Data Store Memory2 : DataStoreMemory  DataStoreName=BSW_EHB_35584err2  ReadBeforeWriteMsg=warning  WriteAfterWriteMsg=warning  WriteAfterReadMsg=warning  ShowAdditionalParam=off  OutDataTypeStr=boolean
      settings: RTWStateStorageClass=ExportedGlobal
  Data Store Memory3 : DataStoreMemory  DataStoreName=BSW_EHB_Ignion  ReadBeforeWriteMsg=warning  WriteAfterWriteMsg=warning  WriteAfterReadMsg=warning  ShowAdditionalParam=off  OutDataTypeStr=boolean
      settings: RTWStateStorageClass=ExportedGlobal
  Data Store Memory6 : DataStoreMemory  DataStoreName=BSW_EHB_35584INT  ReadBeforeWriteMsg=warning  WriteAfterWriteMsg=warning  WriteAfterReadMsg=warning  ShowAdditionalParam=off  OutDataTypeStr=boolean
      settings: RTWStateStorageClass=ExportedGlobal
  Data Store Memory8 : DataStoreMemory  DataStoreName=BSW_EHB_swBrkLED  ReadBeforeWriteMsg=warning  WriteAfterWriteMsg=warning  WriteAfterReadMsg=warning  ShowAdditionalParam=off  OutDataTypeStr=boolean
      settings: RTWStateStorageClass=ExportedGlobal
  Data Store Memory9 : DataStoreMemory  DataStoreName=BSW_EHB_posLiq  ReadBeforeWriteMsg=warning  WriteAfterWriteMsg=warning  WriteAfterReadMsg=warning  ShowAdditionalParam=off  OutDataTypeStr=boolean
      settings: RTWStateStorageClass=ExportedGlobal
  Data Store Read1 : DataStoreRead  DataStoreName=BSW_EHB_35584err1  DataStoreElements=BSW_EHB_35584err1
  Data Store Read10 : DataStoreRead  DataStoreName=BSW_EHB_7189err1  DataStoreElements=BSW_EHB_7189err1
  Data Store Read11 : DataStoreRead  DataStoreName=BSW_EHB_7189err2  DataStoreElements=BSW_EHB_7189err2
  Data Store Read12 : DataStoreRead  DataStoreName=BSW_EHB_HID  DataStoreElements=BSW_EHB_HID
  Data Store Read13 : DataStoreRead  DataStoreName=BSW_EHB_AVH  DataStoreElements=BSW_EHB_AVH
  Data Store Read2 : DataStoreRead  DataStoreName=BSW_EHB_35584err2  DataStoreElements=BSW_EHB_35584err2
  Data Store Read3 : DataStoreRead  DataStoreName=BSW_EHB_Ignion  DataStoreElements=BSW_EHB_Ignion
  Data Store Read6 : DataStoreRead  DataStoreName=BSW_EHB_35584INT  DataStoreElements=BSW_EHB_35584INT
  Data Store Read8 : DataStoreRead  DataStoreName=BSW_EHB_swBrkLED  DataStoreElements=BSW_EHB_swBrkLED
  Data Store Read9 : DataStoreRead  DataStoreName=BSW_EHB_posLiq  DataStoreElements=BSW_EHB_posLiq
  EHB_Ignion : Outport
  EHB_35584err1 : Outport  Port=2
  EHB_35584err2 : Outport  Port=3
  EHB_35584INT : Outport  Port=4
  EHB_swBrkLED : Outport  Port=5
  EHB_posLiq : Outport  Port=6
  EHB_7189err1 : Outport  Port=7
  EHB_7189err2 : Outport  Port=8
  EHB_HID : Outport  Port=9
  EHB_AVH : Outport  Port=10
  wires:
  Data Store Read1/1 -> EHB_35584err1/1
  Data Store Read10/1 -> EHB_7189err1/1
  Data Store Read6/1 -> EHB_35584INT/1
  Data Store Read12/1 -> EHB_HID/1
  Data Store Read2/1 -> EHB_35584err2/1
  Data Store Read8/1 -> EHB_swBrkLED/1
  Data Store Read3/1 -> EHB_Ignion/1
  Data Store Read9/1 -> EHB_posLiq/1
  Data Store Read11/1 -> EHB_7189err2/1
  Data Store Read13/1 -> EHB_AVH/1
